simulink model "MCO_control_scheme"  (R2018b)
settings: Solver=VariableStepAuto  StartTime=0.0  StopTime=50  RelTol=1e-3
values from neighbouring files (symbols this model uses):
  A = [0 1; 0 0 ]    [MCO_library.m]
  Aa = [A Bd*Cd;0 0 Ad]    [MCO_library.m]
  Aa_s = [A Bd*Cd_s;zeros(2) Ad_s]    [MCO_library.m]
  B = [0; 1]    [MCO_library.m]
  Ba = [B;0]    [MCO_library.m]
  Ba_s = [B;0;0]    [MCO_library.m]
  C = [1 0]    [MCO_library.m]
  Ca = [C 0]    [MCO_library.m]
  Ca_s = [C 0 0]    [MCO_library.m]
  des_out = 5    [MCO_library.m]
  G = pinv(B)*Bd    [MCO_library.m]
  G_s = pinv(B)*Bd    [MCO_library.m]
  H = Ht'    [MCO_library.m]
  Ha = Hat'    [MCO_library.m]
  Ha_s = Hat_s'    [MCO_library.m]
  J = 1    [MCO_library.m]
  Ki = Kk_big(1,3)    [MCO_library.m]
  Kk = Kk_big(1,1:2)    [MCO_library.m]
  Nu = X(3,1)/des_out    [MCO_library.m]
  Nx = X(1:2,1)/des_out    [MCO_library.m]
  r = 1    [MCO_library.m]
  w = 5    [MCO_library.m]
undefined symbols (not defined in the file or in its folder): Hb, Hk, K
settings Model: Creator=Francesca  LastModifiedBy=Francesca

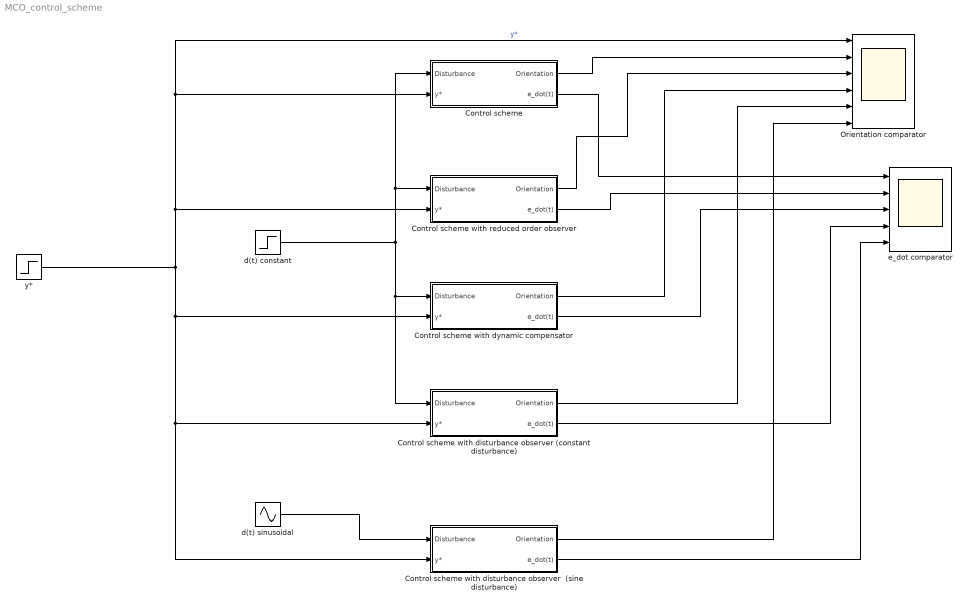
== system MCO_control_scheme ==
  Control scheme : Subsystem  mask{A=A, B=B, C=C, J=J, H=H, K=K, Nx=Nx, Nu=Nu, r=r}
      mask prompts: A "Matrix A"; B "Matrix B"; C "Matrix C"; J "Moment of inertia"; H "Matrix H"; K "Matrix K"; Nx "Filter Nx"; Nu "Filter Nu"; r "Amplitude of cos"
  Control scheme with dynamic compensator : Subsystem  mask{A=A, B=B, C=C, J=J, Hk=Hk, Kk=Kk, Ki=Ki, Nx=Nx, Nu=Nu, Parameter10=r}
      mask prompts: A "Matrix A"; B "Matrix B"; C "Matrix C"; J "Moment of inertia"; Hk "Matrix Hk"; Kk "Matrix Kk"; Ki "Matrix Ki"; Nx "Prefilter Nx"; Nu "Prefilter Nu"; Parameter10 "Amplitude of cos"
  Control scheme with reduced order observer : Subsystem  mask{A=A, B=B, C=C, J=J, Hb=Hb, K=K, Nx=Nx, Nu=Nu, r=r}
      mask prompts: A "Matrix A"; B "Matrix B"; C "Matrix C"; J "Moment of inertia"; Hb "Matrix Hb"; K "Matrix K"; Nx "Prefilter Nx"; Nu "Prefilter Nu"; r "Amplitude of cos"
  Control scheme with disturbance observer  (sine disturbance) : Subsystem  mask{A=A, B=B, C=C, J=J, Aa_s=Aa_s, Ba_s=Ba_s, Ca_s=Ca_s, Ha_s=Ha_s, G_s=G_s, K=K, Nx=Nx, Nu=Nu, r=r}
      mask prompts: A "Matrix A"; B "Matrix B"; C "Matrix C"; J "Moment of inertia"; Aa_s "Matrix Aa_s"; Ba_s "Matrix Ba_s"; Ca_s "Matrix Ca_s"; Ha_s "Matrix Ha_s"; G_s "Matrix G_s"; K "Matrix K"; Nx "Prefilter Nx"; Nu "Prefilter Nu"; r "Amplitude of cos"
  Control scheme with disturbance observer (constant disturbance) : Subsystem  mask{A=A, B=B, C=C, J=J, Aa=Aa, Ba=Ba, Ca=Ca, Ha=Ha, G=G, K=K, Nx=Nx, Nu=Nu, r=r}
      mask prompts: A "Matrix A"; B "Matrix B"; C "Matrix C"; J "Moment of inertia"; Aa "Matrix Aa"; Ba "Matrix Ba"; Ca "Matrix Ca"; Ha "Matrix Ha"; G "Matrix G"; K "Matrix K"; Nx "Prefilter Nx"; Nu "Prefilter Nu"; r "Amplitude of cos"
  Orientation comparator : Scope  NumInputPorts=6
  d(t) constant : Step  Time=0  After=0.5  SampleTime=0
  d(t) sinusoidal : Sin  Amplitude=0.5  Frequency=w  SampleTime=0
  e_dot comparator : Scope  NumInputPorts=5
  y* : Step  Time=0  After=des_out  SampleTime=0
  wires:
  y*/1 -> Orientation comparator/1, Control scheme/2(y*), Control scheme with reduced order observer/2(y*), Control scheme with dynamic compensator/2(y*), Control scheme with disturbance observer  (sine disturbance)/2(y*), Control scheme with disturbance observer (constant disturbance)/2(y*)  "y*"
  Control scheme/1(Orientation) -> Orientation comparator/2
  Control scheme with disturbance observer (constant disturbance)/1(Orientation) -> Orientation comparator/5
  Control scheme with reduced order observer/1(Orientation) -> Orientation comparator/3
  Control scheme with dynamic compensator/1(Orientation) -> Orientation comparator/4
  Control scheme/2(e_dot(t)) -> e_dot comparator/1
  Control scheme with reduced order observer/2(e_dot(t)) -> e_dot comparator/2
  Control scheme with dynamic compensator/2(e_dot(t)) -> e_dot comparator/3
  Control scheme with disturbance observer (constant disturbance)/2(e_dot(t)) -> e_dot comparator/4
  d(t) constant/1 -> Control scheme/1(Disturbance), Control scheme with reduced order observer/1(Disturbance), Control scheme with disturbance observer (constant disturbance)/1(Disturbance), Control scheme with dynamic compensator/1(Disturbance)
  Control scheme with disturbance observer  (sine disturbance)/1(Orientation) -> Orientation comparator/6
  Control scheme with disturbance observer  (sine disturbance)/2(e_dot(t)) -> e_dot comparator/5
  d(t) sinusoidal/1 -> Control scheme with disturbance observer  (sine disturbance)/1(Disturbance)

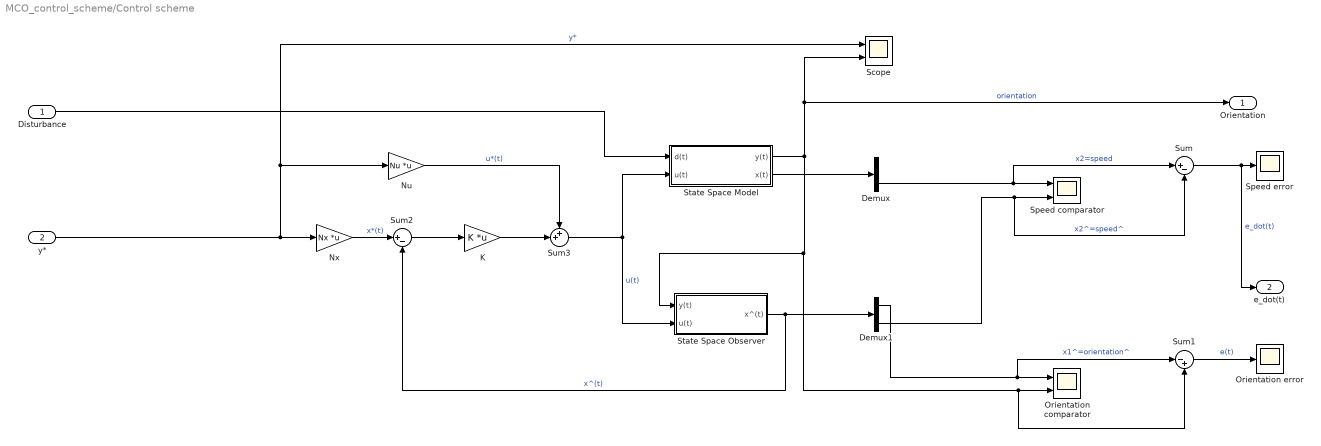
== system MCO_control_scheme/Control scheme ==
  Disturbance : Inport
  y* : Inport  Port=2
  Demux : Demux  Outputs=2
  Demux1 : Demux  Outputs=2
  K : Gain  Gain=K  Multiplication=Matrix(K*u)
  "Nu " : Gain  Gain=Nu  Multiplication=Matrix(K*u)
  Nx : Gain  Gain=Nx  Multiplication=Matrix(K*u)
  "Orientation error " : Scope
  Orientation comparator : Scope  NumInputPorts=2
  Scope : Scope  NumInputPorts=2
  Speed comparator : Scope  NumInputPorts=2
  "Speed error " : Scope
  State Space Model : Subsystem  mask{A=A, B=B, C=C, J=J, r=r}
      mask prompts: A "Matrix A"; B "Matrix B"; C "Matrix C"; J "Moment of inertia"; r "Amplitude of cos"
  State Space Observer : Subsystem  mask{A=A, B=B, C=C, H=H}
      mask prompts: A "Matrix A"; B "Matrix B"; C "Matrix C"; H "Matrix H"
  Sum : Sum  Inputs=|+-
  Sum1 : Sum  Inputs=|-+
  Sum2 : Sum  Inputs=|+-
  Sum3 : Sum  Inputs=++|
  Orientation : Outport
  e_dot(t) : Outport  Port=2
  wires:
  Sum1/1 -> "Orientation error "/1  "e(t)"
  Demux1/2 -> Speed comparator/2, Sum/2  "x2^=speed^"
  y*/1 -> Scope/1, "Nu "/1, Nx/1  "y*"
  "Nu "/1 -> Sum3/1  "u*(t)"
  State Space Model/1(y(t)) -> Orientation/1, Scope/2, Sum1/2, Orientation comparator/2, State Space Observer/1(y(t))  "orientation"
  Sum2/1 -> K/1
  State Space Observer/1(x^(t)) -> Demux1/1, Sum2/2  "x^(t)"
  K/1 -> Sum3/2
  Nx/1 -> Sum2/1  "x*(t)"
  Sum3/1 -> State Space Model/2(u(t)), State Space Observer/2(u(t))  "u(t)"
  Disturbance/1 -> State Space Model/1(d(t))
  Demux1/1 -> Sum1/1, Orientation comparator/1  "x1^=orientation^"
  State Space Model/2(x(t)) -> Demux/1
  Demux/2 -> Sum/1, Speed comparator/1  "x2=speed"
  Sum/1 -> e_dot(t)/1, "Speed error "/1  "e_dot(t)"

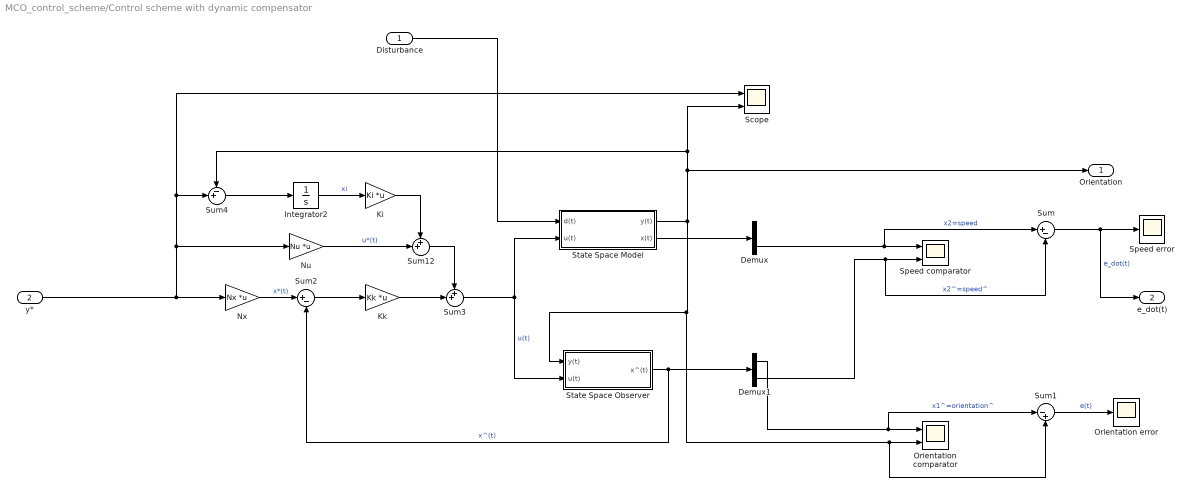
== system MCO_control_scheme/Control scheme with dynamic compensator ==
  Disturbance : Inport
  y* : Inport  Port=2
  Demux : Demux  Outputs=2
  Demux1 : Demux  Outputs=2
  Integrator2 : Integrator  InitialCondition=1
  Ki : Gain  Gain=Ki  Multiplication=Matrix(K*u)
  Kk : Gain  Gain=Kk  Multiplication=Matrix(K*u)
  Nu : Gain  Gain=Nu  Multiplication=Matrix(K*u)
  Nx : Gain  Gain=Nx  Multiplication=Matrix(K*u)
  "Orientation error " : Scope
  Orientation comparator : Scope  NumInputPorts=2
  Scope : Scope  NumInputPorts=2
  Speed comparator : Scope  NumInputPorts=2
  "Speed error " : Scope
  State Space Model : Subsystem  mask{A=A, B=B, C=C, J=J, r=r}
      mask prompts: A "Matrix A"; B "Matrix B"; C "Matrix C"; J "Moment of inertia"; r "Amplitude of cos"
  State Space Observer : Subsystem  mask{A=A, B=B, C=C, Hk=Hk}
      mask prompts: A "Matrix A"; B "Matrix B"; C "Matrix C"; Hk "Matrix Hk"
  Sum : Sum  Inputs=|+-
  Sum1 : Sum  Inputs=|-+
  Sum12 : Sum  Inputs=++|
  Sum2 : Sum  Inputs=|+-
  Sum3 : Sum  Inputs=++|
  Sum4 : Sum  Inputs=-+|
  Orientation : Outport
  e_dot(t) : Outport  Port=2
  wires:
  Sum1/1 -> "Orientation error "/1  "e(t)"
  Demux1/2 -> Speed comparator/2, Sum/2  "x2^=speed^"
  Sum/1 -> e_dot(t)/1, "Speed error "/1  "e_dot(t)"
  Sum2/1 -> Kk/1
  State Space Observer/1(x^(t)) -> Demux1/1, Sum2/2  "x^(t)"
  Kk/1 -> Sum3/2
  Nx/1 -> Sum2/1  "x*(t)"
  Sum3/1 -> State Space Model/2(u(t)), State Space Observer/2(u(t))  "u(t)"
  Disturbance/1 -> State Space Model/1(d(t))
  Demux1/1 -> Sum1/1, Orientation comparator/1  "x1^=orientation^"
  State Space Model/2(x(t)) -> Demux/1
  Demux/2 -> Sum/1, Speed comparator/1  "x2=speed"
  Ki/1 -> Sum12/1
  Sum4/1 -> Integrator2/1
  State Space Model/1(y(t)) -> Orientation/1, Sum4/1, Scope/2, Sum1/2, Orientation comparator/2, State Space Observer/1(y(t))
  y*/1 -> Nx/1, Nu/1, Sum4/2, Scope/1
  Nu/1 -> Sum12/2  "u*(t)"
  Sum12/1 -> Sum3/1
  Integrator2/1 -> Ki/1  "xi"

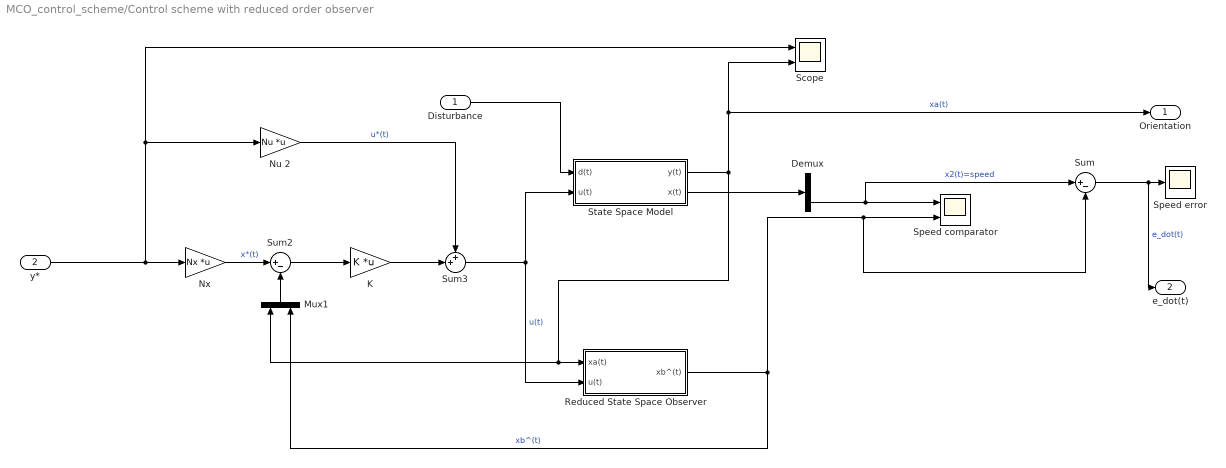
== system MCO_control_scheme/Control scheme with reduced order observer ==
  Disturbance : Inport
  y* : Inport  Port=2
  Demux : Demux  Outputs=2
  K : Gain  Gain=K  Multiplication=Matrix(K*u)
  Mux1 : Mux  Inputs=2
  Nu 2 : Gain  Gain=Nu  Multiplication=Matrix(K*u)
  Nx : Gain  Gain=Nx  Multiplication=Matrix(K*u)
  Reduced State Space Observer : Subsystem  mask{A=A, B=B, C=C, Hb=Hb}
      mask prompts: A "Matrix A"; B "Matrix B"; C "Matrix C"; Hb "Matrix Hb"
  Scope : Scope  NumInputPorts=2
  Speed comparator : Scope  NumInputPorts=2
  "Speed error " : Scope
  State Space Model : Subsystem  mask{A=A, B=B, C=C, J=J, r=r}
      mask prompts: A "Matrix A"; B "Matrix B"; C "Matrix C"; J "Moment of inertia"; r "Amplitude of cos"
  Sum : Sum  Inputs=|+-
  Sum2 : Sum  Inputs=|+-
  Sum3 : Sum  Inputs=++|
  Orientation : Outport
  e_dot(t) : Outport  Port=2
  wires:
  Sum2/1 -> K/1
  Reduced State Space Observer/1(xb^(t)) -> Speed comparator/2, Sum/2, Mux1/2  "xb^(t)"
  K/1 -> Sum3/2
  Nx/1 -> Sum2/1  "x*(t)"
  Sum3/1 -> State Space Model/2(u(t)), Reduced State Space Observer/2(u(t))  "u(t)"
  Disturbance/1 -> State Space Model/1(d(t))
  State Space Model/2(x(t)) -> Demux/1
  Demux/2 -> Speed comparator/1, Sum/1  "x2(t)=speed"
  y*/1 -> Scope/1, Nu 2/1, Nx/1
  Nu 2/1 -> Sum3/1  "u*(t)"
  State Space Model/1(y(t)) -> Orientation/1, Scope/2, Reduced State Space Observer/1(xa(t)), Mux1/1  "xa(t)"
  Mux1/1 -> Sum2/2
  Sum/1 -> e_dot(t)/1, "Speed error "/1  "e_dot(t)"

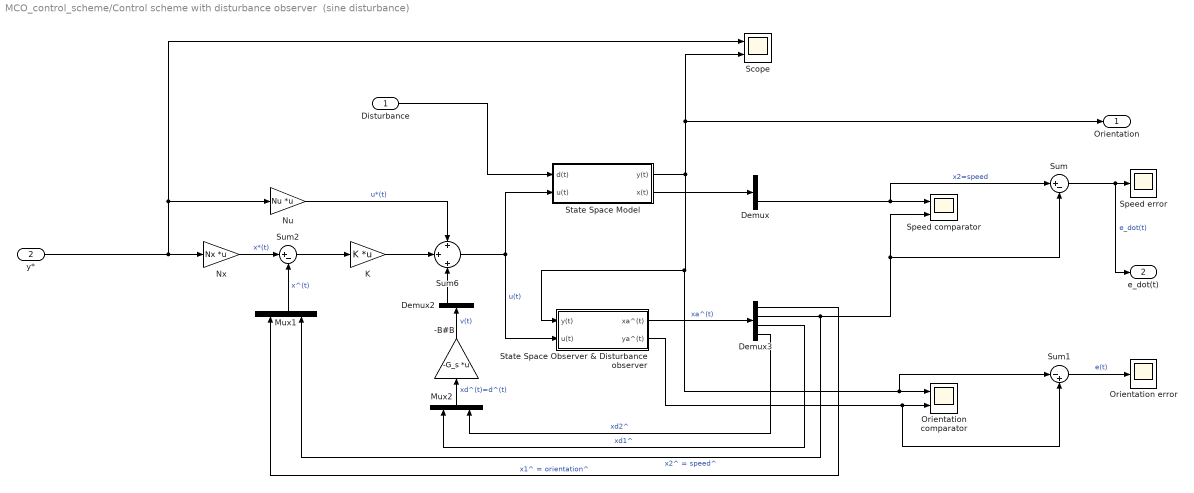
== system MCO_control_scheme/Control scheme with disturbance observer  (sine disturbance) ==
  Disturbance : Inport
  y* : Inport  Port=2
  -B#B : Gain  Gain=-G_s  Multiplication=Matrix(K*u)
  Demux : Demux  Outputs=2
  Demux2 : Demux  Outputs=2
  Demux3 : Demux
  K : Gain  Gain=K  Multiplication=Matrix(K*u)
  Mux1 : Mux  Inputs=2
  Mux2 : Mux  Inputs=2
  Nu : Gain  Gain=Nu  Multiplication=Matrix(K*u)
  Nx : Gain  Gain=Nx  Multiplication=Matrix(K*u)
  "Orientation error " : Scope
  Orientation comparator : Scope  NumInputPorts=2
  Scope : Scope  NumInputPorts=2
  Speed comparator : Scope  NumInputPorts=2
  "Speed error " : Scope
  State Space Model : Subsystem  mask{A=A, B=B, C=C, J=J, r=r}
      mask prompts: A "Matrix A"; B "Matrix B"; C "Matrix C"; J "Moment of inertia"; r "Amplitude of cos"
  "State Space Observer & Disturbance observer " : Subsystem  mask{Aa_s=Aa_s, Ba_s=Ba_s, Ca_s=Ca_s, Ha_s=Ha_s}
      mask prompts: Aa_s "Matrix Aa_a"; Ba_s "Matrix Ba_s"; Ca_s "Matrix Ca_s"; Ha_s "Matrix Ha_s"
  Sum : Sum  Inputs=|+-
  Sum1 : Sum  Inputs=|-+
  Sum2 : Sum  Inputs=|+-
  Sum6 : Sum  Inputs=+|+|+
  Orientation : Outport
  e_dot(t) : Outport  Port=2
  wires:
  Sum1/1 -> "Orientation error "/1  "e(t)"
  Sum2/1 -> K/1
  "State Space Observer & Disturbance observer "/1(xa^(t)) -> Demux3/1  "xa^(t)"
  K/1 -> Sum6/2
  Nx/1 -> Sum2/1  "x*(t)"
  Sum6/1 -> "State Space Observer & Disturbance observer "/2(u(t)), State Space Model/2(u(t))  "u(t)"
  Disturbance/1 -> State Space Model/1(d(t))
  State Space Model/2(x(t)) -> Demux/1
  Demux/2 -> Sum/1, Speed comparator/1  "x2=speed"
  State Space Model/1(y(t)) -> Orientation/1, Scope/2, Sum1/1, Orientation comparator/1, "State Space Observer & Disturbance observer "/1(y(t))
  y*/1 -> Scope/1, Nu/1, Nx/1
  Nu/1 -> Sum6/1  "u*(t)"
  Mux1/1 -> Sum2/2  "x^(t)"
  "State Space Observer & Disturbance observer "/2(ya^(t)) -> Sum1/2, Orientation comparator/2
  Demux3/1 -> Mux1/1  "x1^ = orientation^"
  Sum/1 -> e_dot(t)/1, "Speed error "/1  "e_dot(t)"
  Demux2/1 -> Sum6/3
  -B#B/1 -> Demux2/1  "v(t)"
  Mux2/1 -> -B#B/1  "xd^(t)=d^(t)"
  Demux3/2 -> Sum/2, Speed comparator/2, Mux1/2  "x2^ = speed^"
  Demux3/3 -> Mux2/1  "xd1^"
  Demux3/4 -> Mux2/2  "xd2^"

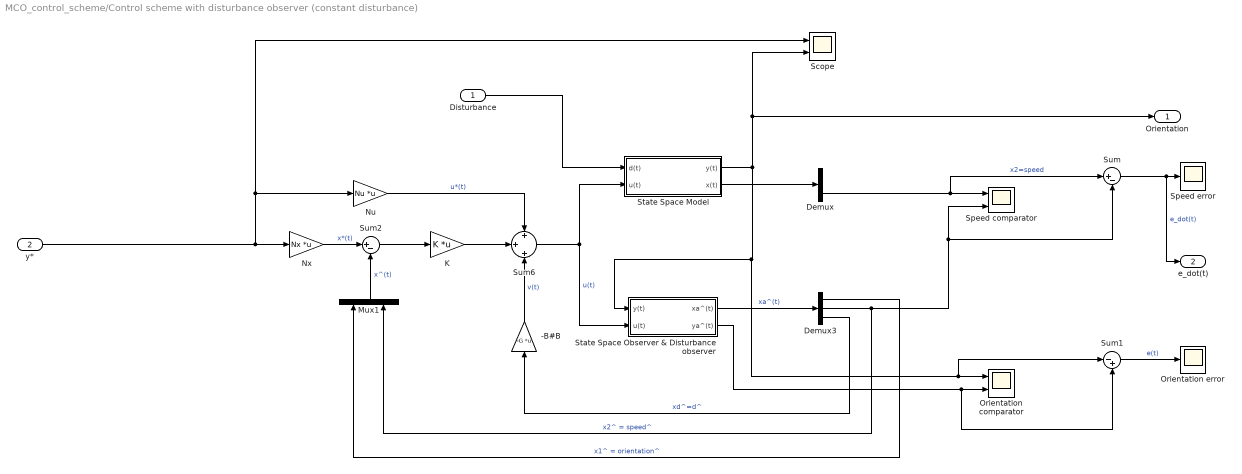
== system MCO_control_scheme/Control scheme with disturbance observer (constant disturbance) ==
  Disturbance : Inport
  y* : Inport  Port=2
  -B#B : Gain  Gain=-G  Multiplication=Matrix(K*u)
  Demux : Demux  Outputs=2
  Demux3 : Demux  Outputs=3
  K : Gain  Gain=K  Multiplication=Matrix(K*u)
  Mux1 : Mux  Inputs=2
  Nu : Gain  Gain=Nu  Multiplication=Matrix(K*u)
  Nx : Gain  Gain=Nx  Multiplication=Matrix(K*u)
  "Orientation error " : Scope
  Orientation comparator : Scope  NumInputPorts=2
  Scope : Scope  NumInputPorts=2
  Speed comparator : Scope  NumInputPorts=2
  "Speed error " : Scope
  State Space Model : Subsystem  mask{A=A, B=B, C=C, J=J, r=r}
      mask prompts: A "Matrix A"; B "Matrix B"; C "Matrix C"; J "Moment of inertia"; r "Amplitude of cos"
  "State Space Observer & Disturbance observer " : Subsystem  mask{Aa=Aa, Ba=Ba, Ca=Ca, Ha=Ha}
      mask prompts: Aa "Matrix Aa"; Ba "Matrix Ba"; Ca "Matrix Ca"; Ha "Matrix Ha"
  Sum : Sum  Inputs=|+-
  Sum1 : Sum  Inputs=|-+
  Sum2 : Sum  Inputs=|+-
  Sum6 : Sum  Inputs=+|+|+
  Orientation : Outport
  e_dot(t) : Outport  Port=2
  wires:
  Sum1/1 -> "Orientation error "/1  "e(t)"
  Sum2/1 -> K/1
  "State Space Observer & Disturbance observer "/1(xa^(t)) -> Demux3/1  "xa^(t)"
  K/1 -> Sum6/2
  Nx/1 -> Sum2/1  "x*(t)"
  Sum6/1 -> "State Space Observer & Disturbance observer "/2(u(t)), State Space Model/2(u(t))  "u(t)"
  Disturbance/1 -> State Space Model/1(d(t))
  State Space Model/2(x(t)) -> Demux/1
  Demux/2 -> Sum/1, Speed comparator/1  "x2=speed"
  State Space Model/1(y(t)) -> Orientation/1, Scope/2, Sum1/1, Orientation comparator/1, "State Space Observer & Disturbance observer "/1(y(t))
  y*/1 -> Scope/1, Nu/1, Nx/1
  Nu/1 -> Sum6/1  "u*(t)"
  Demux3/2 -> Sum/2, Speed comparator/2, Mux1/2  "x2^ = speed^"
  Mux1/1 -> Sum2/2  "x^(t)"
  "State Space Observer & Disturbance observer "/2(ya^(t)) -> Sum1/2, Orientation comparator/2
  Demux3/1 -> Mux1/1  "x1^ = orientation^"
  Demux3/3 -> -B#B/1  "xd^=d^"
  -B#B/1 -> Sum6/3  "v(t)"
  Sum/1 -> e_dot(t)/1, "Speed error "/1  "e_dot(t)"

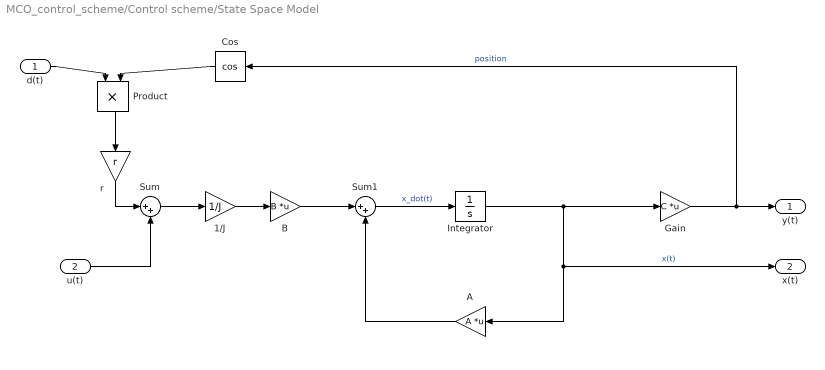
== system MCO_control_scheme/Control scheme/State Space Model ==
  d(t) : Inport
  u(t) : Inport  Port=2
  1/J : Gain  Gain=1/J
  A : Gain  Gain=A  Multiplication=Matrix(K*u)
  B : Gain  Gain=B  Multiplication=Matrix(K*u)
  Cos : Trigonometry  Operator=cos
  Gain : Gain  Gain=C  Multiplication=Matrix(K*u)
  Integrator : Integrator  InitialCondition=1
  Product : Product
  Sum : Sum  Inputs=|++
  Sum1 : Sum  Inputs=|++
  r : Gain  Gain=r
  y(t) : Outport
  x(t) : Outport  Port=2
  wires:
  u(t)/1 -> Sum/2
  Integrator/1 -> Gain/1, A/1, x(t)/1  "x(t)"
  A/1 -> Sum1/2
  Sum1/1 -> Integrator/1  "x_dot(t)"
  B/1 -> Sum1/1
  1/J/1 -> B/1
  Sum/1 -> 1/J/1
  Gain/1 -> Cos/1, y(t)/1  "position"
  Cos/1 -> Product/2
  Product/1 -> r/1
  d(t)/1 -> Product/1
  r/1 -> Sum/1

== system MCO_control_scheme/Control scheme/State Space Observer ==
  y(t) : Inport
  u(t) : Inport  Port=2
  A : Gain  Gain=A  Multiplication=Matrix(K*u)
  B : Gain  Gain=B  Multiplication=Matrix(K*u)
  C : Gain  Gain=C  Multiplication=Matrix(K*u)
  H : Gain  Gain=H  Multiplication=Matrix(K*u)
  Integrator : Integrator
  Sum : Sum  Inputs=-+|
  Sum1 : Sum  Inputs=+|+|+
  x^(t) : Outport
  wires:
  u(t)/1 -> B/1
  Integrator/1 -> C/1, x^(t)/1, A/1  "x^(t)"
  Sum1/1 -> Integrator/1  "x_hat_dot(t)"
  y(t)/1 -> Sum/2
  C/1 -> Sum/1
  Sum/1 -> H/1
  H/1 -> Sum1/1
  B/1 -> Sum1/2
  A/1 -> Sum1/3

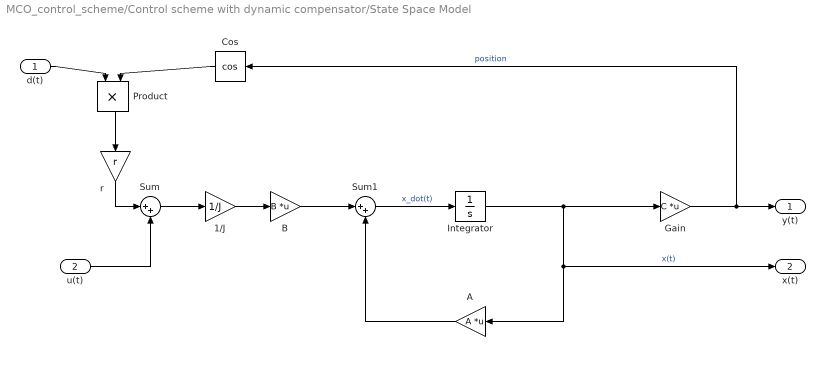
== system MCO_control_scheme/Control scheme with dynamic compensator/State Space Model ==
  d(t) : Inport
  u(t) : Inport  Port=2
  1/J : Gain  Gain=1/J
  A : Gain  Gain=A  Multiplication=Matrix(K*u)
  B : Gain  Gain=B  Multiplication=Matrix(K*u)
  Cos : Trigonometry  Operator=cos
  Gain : Gain  Gain=C  Multiplication=Matrix(K*u)
  Integrator : Integrator  InitialCondition=1
  Product : Product
  Sum : Sum  Inputs=|++
  Sum1 : Sum  Inputs=|++
  r : Gain  Gain=r
  y(t) : Outport
  x(t) : Outport  Port=2
  wires:
  Product/1 -> r/1
  B/1 -> Sum1/1
  Gain/1 -> Cos/1, y(t)/1  "position"
  1/J/1 -> B/1
  A/1 -> Sum1/2
  Integrator/1 -> Gain/1, A/1, x(t)/1  "x(t)"
  Sum1/1 -> Integrator/1  "x_dot(t)"
  u(t)/1 -> Sum/2
  r/1 -> Sum/1
  Sum/1 -> 1/J/1
  d(t)/1 -> Product/1
  Cos/1 -> Product/2

== system MCO_control_scheme/Control scheme with dynamic compensator/State Space Observer ==
  y(t) : Inport
  u(t) : Inport  Port=2
  A : Gain  Gain=A  Multiplication=Matrix(K*u)
  B : Gain  Gain=B  Multiplication=Matrix(K*u)
  C : Gain  Gain=C  Multiplication=Matrix(K*u)
  Hk : Gain  Gain=Hk  Multiplication=Matrix(K*u)
  Integrator : Integrator
  Sum : Sum  Inputs=-+|
  Sum1 : Sum  Inputs=+|+|+
  x^(t) : Outport
  wires:
  u(t)/1 -> B/1
  Integrator/1 -> C/1, x^(t)/1, A/1  "x^(t)"
  Sum1/1 -> Integrator/1  "x_hat_dot(t)"
  y(t)/1 -> Sum/2
  C/1 -> Sum/1
  Sum/1 -> Hk/1
  Hk/1 -> Sum1/1
  B/1 -> Sum1/2
  A/1 -> Sum1/3

== system MCO_control_scheme/Control scheme with reduced order observer/Reduced State Space Observer ==
  note: eta^(t)
  xa(t) : Inport
  u(t) : Inport  Port=2
  Integrator : Integrator
  Sum : Sum  Inputs=+|+||
  Sum1 : Sum  Inputs=-|+|-
  hb : Gain  Gain=Hb
  hb1 : Gain  Gain=Hb
  hb2 : Gain  Gain=Hb
  xb^(t) : Outport
  wires:
  hb1/1 -> Sum1/3
  hb2/1 -> Sum1/1
  Integrator/1 -> Sum/2, hb1/1
  Sum1/1 -> Integrator/1  "eta_hat_dot(t)"
  hb/1 -> hb2/1, Sum/1
  Sum/1 -> xb^(t)/1
  xa(t)/1 -> hb/1
  u(t)/1 -> Sum1/2

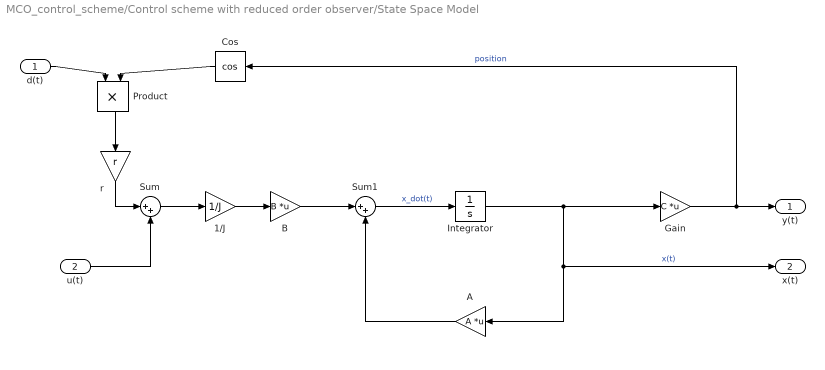
== system MCO_control_scheme/Control scheme with reduced order observer/State Space Model ==
  d(t) : Inport
  u(t) : Inport  Port=2
  1/J : Gain  Gain=1/J
  A : Gain  Gain=A  Multiplication=Matrix(K*u)
  B : Gain  Gain=B  Multiplication=Matrix(K*u)
  Cos : Trigonometry  Operator=cos
  Gain : Gain  Gain=C  Multiplication=Matrix(K*u)
  Integrator : Integrator  InitialCondition=1
  Product : Product
  Sum : Sum  Inputs=|++
  Sum1 : Sum  Inputs=|++
  r : Gain  Gain=r
  y(t) : Outport
  x(t) : Outport  Port=2
  wires:
  Product/1 -> r/1
  B/1 -> Sum1/1
  Gain/1 -> Cos/1, y(t)/1  "position"
  1/J/1 -> B/1
  A/1 -> Sum1/2
  Integrator/1 -> Gain/1, A/1, x(t)/1  "x(t)"
  Sum1/1 -> Integrator/1  "x_dot(t)"
  u(t)/1 -> Sum/2
  r/1 -> Sum/1
  Sum/1 -> 1/J/1
  d(t)/1 -> Product/1
  Cos/1 -> Product/2

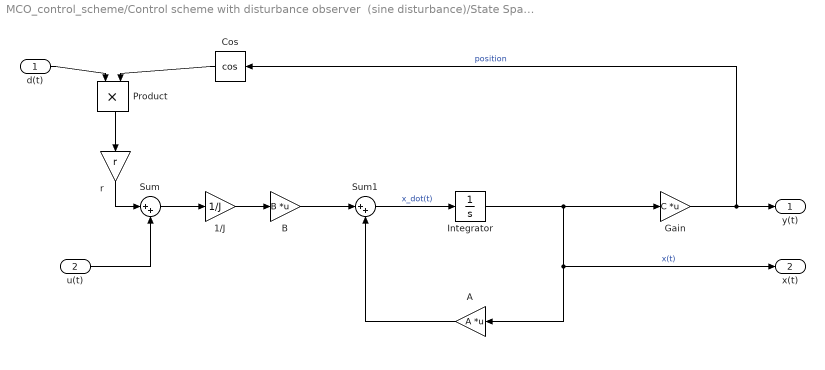
== system MCO_control_scheme/Control scheme with disturbance observer  (sine disturbance)/State Space Model ==
  d(t) : Inport
  u(t) : Inport  Port=2
  1/J : Gain  Gain=1/J
  A : Gain  Gain=A  Multiplication=Matrix(K*u)
  B : Gain  Gain=B  Multiplication=Matrix(K*u)
  Cos : Trigonometry  Operator=cos
  Gain : Gain  Gain=C  Multiplication=Matrix(K*u)
  Integrator : Integrator  InitialCondition=1
  Product : Product
  Sum : Sum  Inputs=|++
  Sum1 : Sum  Inputs=|++
  r : Gain  Gain=r
  y(t) : Outport
  x(t) : Outport  Port=2
  wires:
  Product/1 -> r/1
  B/1 -> Sum1/1
  Gain/1 -> Cos/1, y(t)/1  "position"
  1/J/1 -> B/1
  A/1 -> Sum1/2
  Integrator/1 -> Gain/1, A/1, x(t)/1  "x(t)"
  Sum1/1 -> Integrator/1  "x_dot(t)"
  u(t)/1 -> Sum/2
  r/1 -> Sum/1
  Sum/1 -> 1/J/1
  d(t)/1 -> Product/1
  Cos/1 -> Product/2

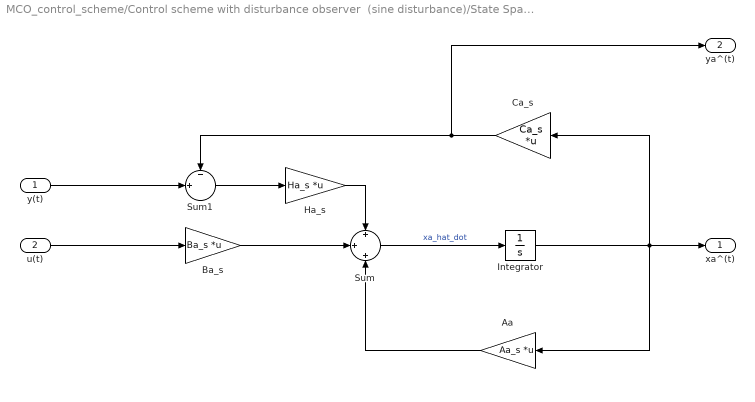
== system MCO_control_scheme/Control scheme with disturbance observer  (sine disturbance)/State Space Observer & Disturbance observer  ==
  y(t) : Inport
  u(t) : Inport  Port=2
  Aa : Gain  Gain=Aa_s  Multiplication=Matrix(K*u)
  Ba_s : Gain  Gain=Ba_s  Multiplication=Matrix(K*u)
  Ca_s : Gain  Gain=Ca_s  Multiplication=Matrix(K*u)
  Ha_s : Gain  Gain=Ha_s  Multiplication=Matrix(K*u)
  Integrator : Integrator
  Sum : Sum  Inputs=+|+|+
  Sum1 : Sum  Inputs=-|+||
  xa^(t) : Outport
  ya^(t) : Outport  Port=2
  wires:
  Ba_s/1 -> Sum/2
  Aa/1 -> Sum/3
  Ha_s/1 -> Sum/1
  Integrator/1 -> Ca_s/1, xa^(t)/1, Aa/1
  y(t)/1 -> Sum1/2
  Sum1/1 -> Ha_s/1
  u(t)/1 -> Ba_s/1
  Ca_s/1 -> ya^(t)/1, Sum1/1
  Sum/1 -> Integrator/1  "xa_hat_dot"

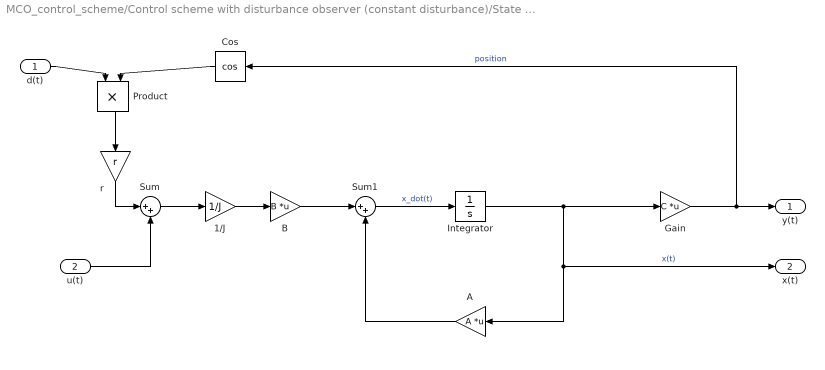
== system MCO_control_scheme/Control scheme with disturbance observer (constant disturbance)/State Space Model ==
  d(t) : Inport
  u(t) : Inport  Port=2
  1/J : Gain  Gain=1/J
  A : Gain  Gain=A  Multiplication=Matrix(K*u)
  B : Gain  Gain=B  Multiplication=Matrix(K*u)
  Cos : Trigonometry  Operator=cos
  Gain : Gain  Gain=C  Multiplication=Matrix(K*u)
  Integrator : Integrator  InitialCondition=1
  Product : Product
  Sum : Sum  Inputs=|++
  Sum1 : Sum  Inputs=|++
  r : Gain  Gain=r
  y(t) : Outport
  x(t) : Outport  Port=2
  wires:
  Product/1 -> r/1
  B/1 -> Sum1/1
  Gain/1 -> Cos/1, y(t)/1  "position"
  1/J/1 -> B/1
  A/1 -> Sum1/2
  Integrator/1 -> Gain/1, A/1, x(t)/1  "x(t)"
  Sum1/1 -> Integrator/1  "x_dot(t)"
  u(t)/1 -> Sum/2
  r/1 -> Sum/1
  Sum/1 -> 1/J/1
  d(t)/1 -> Product/1
  Cos/1 -> Product/2

== system MCO_control_scheme/Control scheme with disturbance observer (constant disturbance)/State Space Observer & Disturbance observer  ==
  y(t) : Inport
  u(t) : Inport  Port=2
  Aa : Gain  Gain=Aa  Multiplication=Matrix(K*u)
  Ba : Gain  Gain=Ba  Multiplication=Matrix(K*u)
  Ca : Gain  Gain=Ca  Multiplication=Matrix(K*u)
  Ha : Gain  Gain=Ha  Multiplication=Matrix(K*u)
  Integrator : Integrator
  Sum : Sum  Inputs=+|+|+
  Sum1 : Sum  Inputs=-|+||
  xa^(t) : Outport
  ya^(t) : Outport  Port=2
  wires:
  Ba/1 -> Sum/2
  Aa/1 -> Sum/3
  Ha/1 -> Sum/1
  Integrator/1 -> Ca/1, xa^(t)/1, Aa/1
  y(t)/1 -> Sum1/2
  Sum1/1 -> Ha/1
  u(t)/1 -> Ba/1
  Ca/1 -> ya^(t)/1, Sum1/1
  Sum/1 -> Integrator/1  "xa_hat_dot"
